simulink model "senoidetestar"  (R2020a)
settings: Solver=ode4  StartTime=0.0  StopTime=10.0  FixedStep=0.001  RelTol=1e-3
values from neighbouring files (symbols this model uses):
  K = yinf/A    [alg4.m]    (also in alg7.m = 10^(pontos(1)/20); ordem1area.m = y/A; ordem1areaneperiano.m = y/A)
  tau = a0/yinf -1    [alg5.m]    (also in alg6.m = 1/a; alg7.m = 1/wc; ordem1area.m = Ao/y; ordem1areaneperiano.m = 1/a)
settings Model: Creator=andre  LastModifiedBy=andre

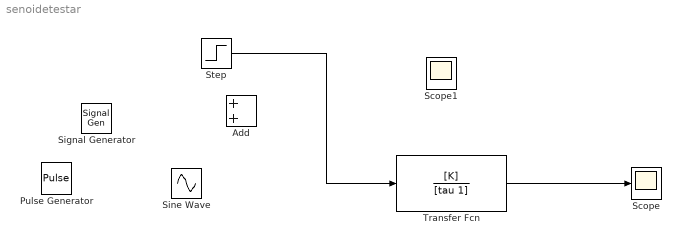
== system senoidetestar ==
  Add : Sum
  Pulse Generator : DiscretePulseGenerator  PulseType=Time based  Period=10  PulseWidth=5
  Scope : Scope
  Scope1 : Scope
  Signal Generator : SignalGenerator  Frequency=1.57  Units=rad/sec
  Sine Wave : Sin  SampleTime=0
  Step : Step  After=2  SampleTime=0
  Transfer Fcn : TransferFcn  Numerator=[K]  Denominator=[tau 1]
  wires:
  Transfer Fcn/1 -> Scope/1
  Step/1 -> Transfer Fcn/1
